simulink model "Pulsar_KTR_UBR"  (R2023b)
settings: Solver=VariableStepAuto  StartTime=0.0  StopTime=10  RelTol=1e-3
values from neighbouring files (symbols this model uses):
  itkip = [2411 2135 2015 2000 2055 2098 1860 1788 1659 1468 1423 1334 ... (23 elements, 23x1)]    [matlabubr.mat]
  zamanp = [0.1 0.2 0.3 0.4 0.5 1 1.5 2 2.5 3 3.25 3.35 ... (23 elements, 23x1)]    [matlabubr.mat]
undefined symbols (not defined in the file or in its folder): magnitude
libraries: simulink x1
settings Model: Creator=atzml  LastModifiedBy=atzml
settings OptimizationCC: BlockReduction=off  DefaultParameterBehavior=Inlined  BufferReuse=off

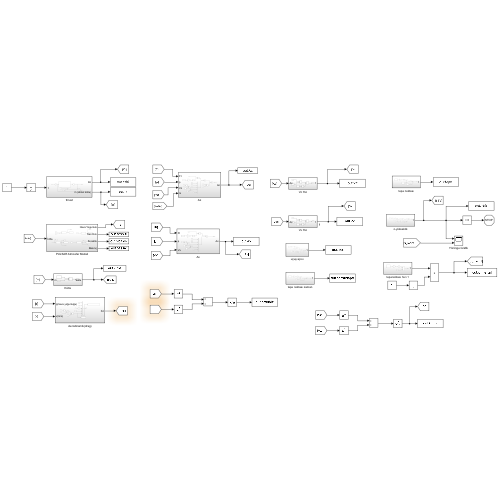
[thumbnail: Simulink's stored preview of the top-level diagram]
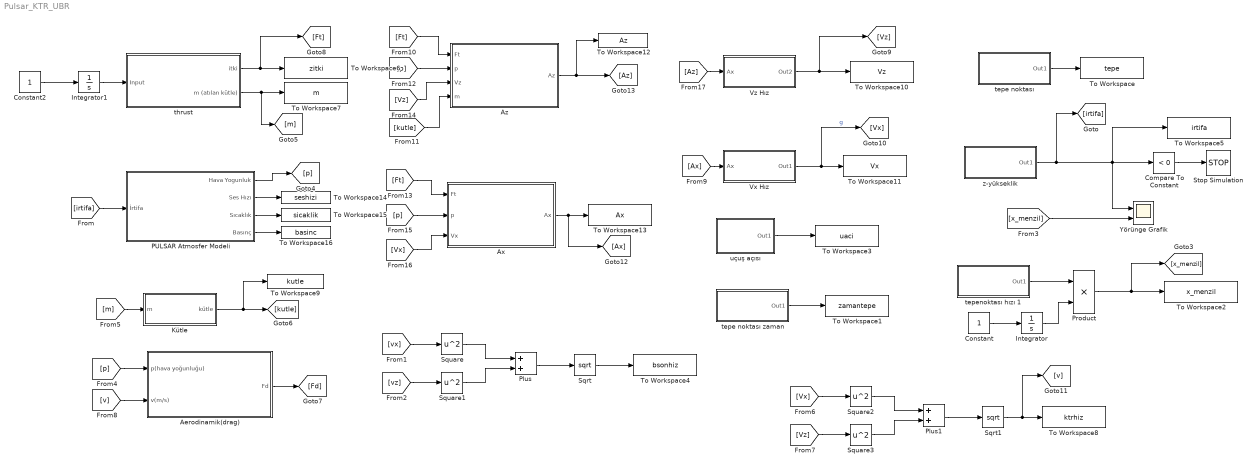
== system Pulsar_KTR_UBR ==
  Aerodinamik(drag) : Subsystem
  Ax : Subsystem
  Az : Subsystem
  Compare To Constant : simulink/Logic and Bit Operations/Compare To Constant  relop=<  const=0  OutDataTypeStr=boolean
  Constant : Constant
  Constant2 : Constant
  Integrator : Integrator
  Integrator1 : Integrator
  Kütle : Subsystem
  PULSAR Atmosfer Modeli : Subsystem
  Plus : Sum
  Plus1 : Sum
  Product : Product
  Sqrt : Sqrt
  Sqrt1 : Sqrt
  Square{,1..3} (4 alike) : Math  Operator=square
  Stop Simulation : Stop
  To Workspace : ToWorkspace  VariableName=tepe  SaveFormat=Timeseries  SampleTime=-1
  To Workspace1 : ToWorkspace  VariableName=zamantepe  SaveFormat=Timeseries  SampleTime=-1
  To Workspace10 : ToWorkspace  VariableName=Vz  SaveFormat=Timeseries  SampleTime=-1
  To Workspace11 : ToWorkspace  VariableName=Vx  SaveFormat=Timeseries  SampleTime=-1
  To Workspace12 : ToWorkspace  VariableName=Az  SaveFormat=Timeseries  SampleTime=-1
  To Workspace13 : ToWorkspace  VariableName=Ax  SaveFormat=Timeseries  SampleTime=-1
  To Workspace14 : ToWorkspace  VariableName=seshizi  SaveFormat=Timeseries  SampleTime=-1
  To Workspace15 : ToWorkspace  VariableName=sicaklik  SaveFormat=Timeseries  SampleTime=-1
  To Workspace16 : ToWorkspace  VariableName=basinc  SaveFormat=Timeseries  SampleTime=-1
  To Workspace2 : ToWorkspace  VariableName=x_menzil  SaveFormat=Timeseries  SampleTime=-1
  To Workspace3 : ToWorkspace  VariableName=uaci  SaveFormat=Timeseries  SampleTime=-1
  To Workspace4 : ToWorkspace  VariableName=bsonhiz  SaveFormat=Timeseries  SampleTime=-1
  To Workspace5 : ToWorkspace  VariableName=irtifa  SaveFormat=Timeseries  SampleTime=-1
  To Workspace6 : ToWorkspace  VariableName=zitki  SampleTime=-1
  To Workspace7 : ToWorkspace  VariableName=m  SaveFormat=Timeseries  SampleTime=-1
  To Workspace8 : ToWorkspace  VariableName=ktrhiz  SaveFormat=Timeseries  SampleTime=-1
  To Workspace9 : ToWorkspace  VariableName=kutle  SaveFormat=Timeseries  SampleTime=-1
  Vx Hız : Subsystem
  Vz Hız : Subsystem
  Yörünge Grafik : Scope  NumInputPorts=2
  tepe noktası : Subsystem
  tepe noktası zaman : Subsystem
  tepenoktası hızı 1 : Subsystem
  thrust : Subsystem
  uçuş açısı : Subsystem
  z-yükseklik : Subsystem
  wires:
  Compare To Constant/1 -> Stop Simulation/1
  Plus/1 -> Sqrt/1
  Constant/1 -> Integrator/1
  Square/1 -> Plus/1
  tepe noktası/1(Out1) -> To Workspace/1
  [x_menzil] -> Yörünge Grafik/2
  z-yükseklik/1(Out1) -> [irtifa], Yörünge Grafik/1, Compare To Constant/1, To Workspace5/1
  Integrator/1 -> Product/2
  Sqrt/1 -> To Workspace4/1
  Product/1 -> [x_menzil], To Workspace2/1
  tepenoktası hızı 1/1(Out1) -> Product/1
  [vz] -> Square1/1
  [vx] -> Square/1
  Square1/1 -> Plus/2
  tepe noktası zaman/1(Out1) -> To Workspace1/1
  uçuş açısı/1(Out1) -> To Workspace3/1
  [irtifa] -> PULSAR Atmosfer Modeli/1(İrtifa)
  PULSAR Atmosfer Modeli/1(Hava Yogunluk) -> [p]
  [p] -> Aerodinamik(drag)/1(p(hava yoğunluğu))
  [v] -> Aerodinamik(drag)/2(v(m/s))
  Aerodinamik(drag)/1(Fd) -> [Fd]
  thrust/2(m (atılan kütle)) -> [m], To Workspace7/1
  thrust/1(itki) -> [Ft], To Workspace6/1
  Constant2/1 -> Integrator1/1
  [m] -> Kütle/1(m)
  Kütle/1(kütle) -> To Workspace9/1, [kutle]
  Integrator1/1 -> thrust/1(Input)
  Vx Hız/1(Out1) -> To Workspace11/1, [Vx]  "g"
  Vz Hız/1(Out2) -> To Workspace10/1, [Vz]
  [Ft] -> Az/1(Ft)
  [kutle] -> Az/4(m)
  [p] -> Az/2(p)
  [p] -> Ax/2(p)
  [Ft] -> Ax/1(Ft)
  [Vz] -> Az/3(Vz)
  [Vx] -> Ax/3(Vx)
  Plus1/1 -> Sqrt1/1
  Sqrt1/1 -> [v], To Workspace8/1
  [Vx] -> Square2/1
  [Vz] -> Square3/1
  Square3/1 -> Plus1/2
  Square2/1 -> Plus1/1
  Ax/1(Ax) -> To Workspace13/1, [Ax]
  [Ax] -> Vx Hız/1(Ax)
  Az/1(Az) -> To Workspace12/1, [Az]
  [Az] -> Vz Hız/1(Ax)
  PULSAR Atmosfer Modeli/2(Ses Hızı) -> To Workspace14/1
  PULSAR Atmosfer Modeli/3(Sıcaklık) -> To Workspace15/1
  PULSAR Atmosfer Modeli/4(Basınç) -> To Workspace16/1

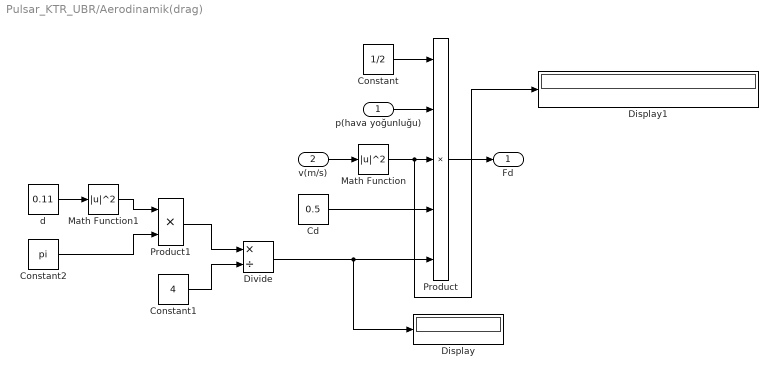
== system Pulsar_KTR_UBR/Aerodinamik(drag) ==
  p(hava yoğunluğu) : Inport
  v(m/s) : Inport  Port=2
  Cd : Constant  Value=0.5
  Constant : Constant  Value=1/2
  Constant1 : Constant  Value=4
  Constant2 : Constant  Value=pi
  Display : Display
  Display1 : Display
  Divide : Product  Inputs=*/
  Math Function : Math  Operator=magnitude^2
  Math Function1 : Math  Operator=magnitude^2
  Product : Product  Inputs=5
  Product1 : Product
  d : Constant  Value=0.11
  Fd : Outport
  wires:
  v(m/s)/1 -> Math Function/1
  Constant/1 -> Product/1
  p(hava yoğunluğu)/1 -> Product/2
  Math Function/1 -> Display1/1, Product/3
  Product/1 -> Fd/1
  Cd/1 -> Product/4
  Divide/1 -> Display/1, Product/5
  d/1 -> Math Function1/1
  Constant2/1 -> Product1/2
  Math Function1/1 -> Product1/1
  Product1/1 -> Divide/1
  Constant1/1 -> Divide/2

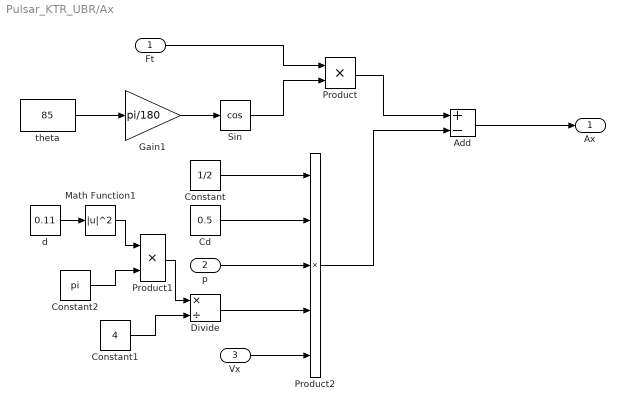
== system Pulsar_KTR_UBR/Ax ==
  Ft : Inport
  p : Inport  Port=2
  Vx : Inport  Port=3
  Add : Sum  Inputs=+-
  Cd : Constant  Value=0.5
  Constant : Constant  Value=1/2
  Constant1 : Constant  Value=4
  Constant2 : Constant  Value=pi
  Divide : Product  Inputs=*/
  Gain1 : Gain  Gain=pi/180
  Math Function1 : Math  Operator=magnitude^2
  Product : Product
  Product1 : Product
  Product2 : Product  Inputs=5
  Sin : Trigonometry  Operator=cos
  d : Constant  Value=0.11
  theta : Constant  Value=85
  Ax : Outport
  wires:
  Gain1/1 -> Sin/1
  theta/1 -> Gain1/1
  Ft/1 -> Product/1
  Sin/1 -> Product/2
  d/1 -> Math Function1/1
  Product1/1 -> Divide/1
  Constant1/1 -> Divide/2
  Constant2/1 -> Product1/2
  Math Function1/1 -> Product1/1
  Product/1 -> Add/1
  Constant/1 -> Product2/1
  Cd/1 -> Product2/2
  p/1 -> Product2/3
  Divide/1 -> Product2/4
  Product2/1 -> Add/2
  Vx/1 -> Product2/5
  Add/1 -> Ax/1

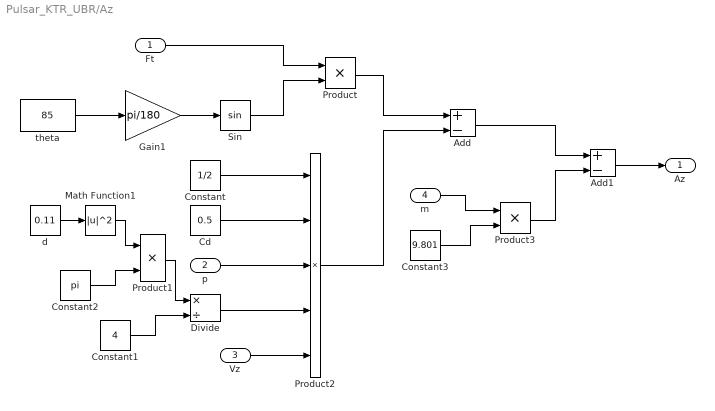
== system Pulsar_KTR_UBR/Az ==
  Ft : Inport
  p : Inport  Port=2
  Vz : Inport  Port=3
  m : Inport  Port=4
  Add : Sum  Inputs=+-
  Add1 : Sum  Inputs=+-
  Cd : Constant  Value=0.5
  Constant : Constant  Value=1/2
  Constant1 : Constant  Value=4
  Constant2 : Constant  Value=pi
  Constant3 : Constant  Value=9.801
  Divide : Product  Inputs=*/
  Gain1 : Gain  Gain=pi/180
  Math Function1 : Math  Operator=magnitude^2
  Product : Product
  Product1 : Product
  Product2 : Product  Inputs=5
  Product3 : Product
  Sin : Trigonometry
  d : Constant  Value=0.11
  theta : Constant  Value=85
  Az : Outport
  wires:
  Gain1/1 -> Sin/1
  theta/1 -> Gain1/1
  Ft/1 -> Product/1
  Sin/1 -> Product/2
  d/1 -> Math Function1/1
  Product1/1 -> Divide/1
  Constant1/1 -> Divide/2
  Constant2/1 -> Product1/2
  Math Function1/1 -> Product1/1
  Product/1 -> Add/1
  Constant/1 -> Product2/1
  Cd/1 -> Product2/2
  p/1 -> Product2/3
  Divide/1 -> Product2/4
  Product2/1 -> Add/2
  Vz/1 -> Product2/5
  m/1 -> Product3/1
  Constant3/1 -> Product3/2
  Add/1 -> Add1/1
  Product3/1 -> Add1/2
  Add1/1 -> Az/1

== system Pulsar_KTR_UBR/Kütle ==
  m : Inport
  Add : Sum
  Constant : Constant  Value=21.649
  kütle : Outport
  wires:
  m/1 -> Add/2
  Constant/1 -> Add/1
  Add/1 -> kütle/1

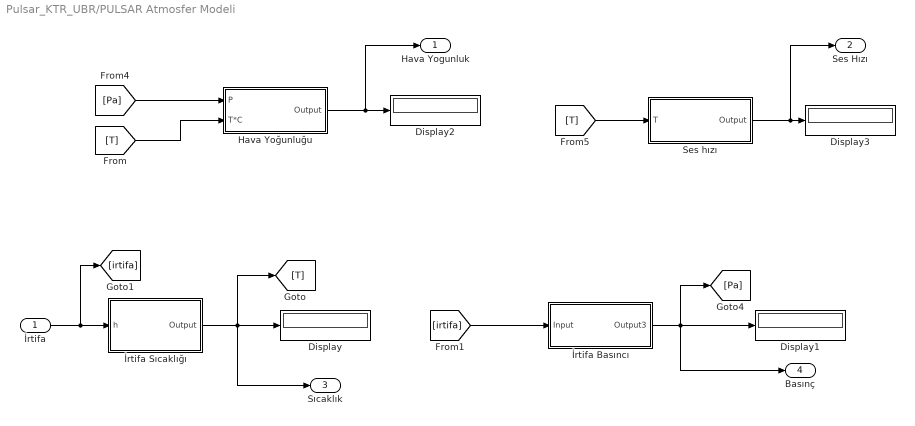
== system Pulsar_KTR_UBR/PULSAR Atmosfer Modeli ==
  İrtifa : Inport
  Display{,1..3} (4 alike) : Display
  Hava Yoğunluğu : Subsystem
  Ses hızı : Subsystem
  İrtifa Basıncı : Subsystem
  İrtifa Sıcaklığı : Subsystem
  Hava Yogunluk : Outport
  Ses Hızı : Outport  Port=2
  Sıcaklık : Outport  Port=3
  Basınç : Outport  Port=4
  wires:
  [irtifa] -> İrtifa Basıncı/1(Input)
  Hava Yoğunluğu/1(Output) -> Hava Yogunluk/1, Display2/1
  İrtifa/1 -> [irtifa], İrtifa Sıcaklığı/1(h)
  Ses hızı/1(Output) -> Ses Hızı/1, Display3/1
  İrtifa Sıcaklığı/1(Output) -> Sıcaklık/1, Display/1, [T]
  [Pa] -> Hava Yoğunluğu/1(P)
  İrtifa Basıncı/1(Output3) -> Basınç/1, Display1/1, [Pa]
  [T] -> Ses hızı/1(T)
  [T] -> Hava Yoğunluğu/2(T*C)

== system Pulsar_KTR_UBR/Vx Hız ==
  Ax : Inport
  Add : Sum
  Constant : Constant
  Integrator : Integrator
  Product : Product
  V0 : Constant  Value=2
  Out1 : Outport
  wires:
  V0/1 -> Add/2
  Ax/1 -> Add/1
  Add/1 -> Product/1
  Constant/1 -> Integrator/1
  Integrator/1 -> Product/2
  Product/1 -> Out1/1

== system Pulsar_KTR_UBR/Vz Hız ==
  Ax : Inport
  Add : Sum
  Constant : Constant
  Integrator : Integrator
  Product : Product
  V0 : Constant  Value=2
  Out2 : Outport
  wires:
  Constant/1 -> Integrator/1
  Product/1 -> Out2/1
  V0/1 -> Add/2
  Ax/1 -> Add/1
  Add/1 -> Product/1
  Integrator/1 -> Product/2

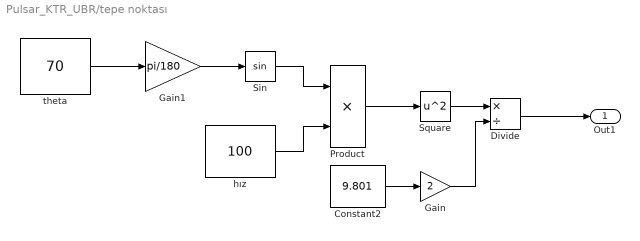
== system Pulsar_KTR_UBR/tepe noktası ==
  Constant2 : Constant  Value=9.801
  Divide : Product  Inputs=*/
  Gain : Gain  Gain=2
  Gain1 : Gain  Gain=pi/180
  Product : Product
  Sin : Trigonometry
  Square : Math  Operator=square
  hız : Constant  Value=100
  theta : Constant  Value=70
  Out1 : Outport
  wires:
  Sin/1 -> Product/1
  hız/1 -> Product/2
  Product/1 -> Square/1
  Square/1 -> Divide/1
  Constant2/1 -> Gain/1
  Gain/1 -> Divide/2
  Divide/1 -> Out1/1
  theta/1 -> Gain1/1
  Gain1/1 -> Sin/1

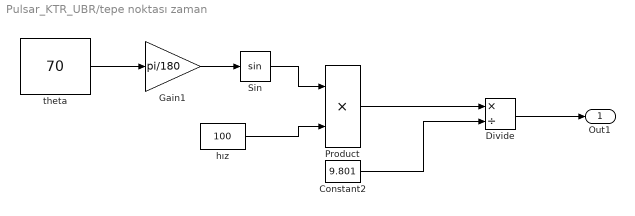
== system Pulsar_KTR_UBR/tepe noktası zaman ==
  Constant2 : Constant  Value=9.801
  Divide : Product  Inputs=*/
  Gain1 : Gain  Gain=pi/180
  Product : Product
  Sin : Trigonometry
  hız : Constant  Value=100
  theta : Constant  Value=70
  Out1 : Outport
  wires:
  Divide/1 -> Out1/1
  hız/1 -> Product/2
  Product/1 -> Divide/1
  Constant2/1 -> Divide/2
  Sin/1 -> Product/1
  Gain1/1 -> Sin/1
  theta/1 -> Gain1/1

== system Pulsar_KTR_UBR/tepenoktası hızı 1 ==
  Gain1 : Gain  Gain=pi/180
  Product : Product
  Sin : Trigonometry  Operator=cos
  hız : Constant  Value=100
  theta : Constant  Value=70
  Out1 : Outport
  wires:
  theta/1 -> Gain1/1
  Gain1/1 -> Sin/1
  hız/1 -> Product/2
  Sin/1 -> Product/1
  Product/1 -> Out1/1  "yatay hız"

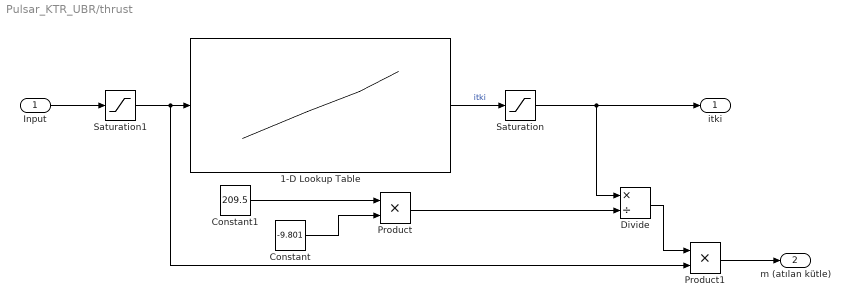
== system Pulsar_KTR_UBR/thrust ==
  Input : Inport
  1-D Lookup Table : Lookup_n-D  NumberOfTableDimensions=1  BreakpointsForDimension1=zamanp  Table=itkip  InternalRulePriority=Speed  RndMeth=Simplest
  Constant : Constant  Value=-9.801
  Constant1 : Constant  Value=209.5
  Divide : Product  Inputs=*/
  Product : Product
  Product1 : Product
  Saturation : Saturate  UpperLimit=3700  LowerLimit=0
  Saturation1 : Saturate  UpperLimit=6.5  LowerLimit=0
  itki : Outport
  m (atılan kütle) : Outport  Port=2
  wires:
  Constant/1 -> Product/2
  Constant1/1 -> Product/1
  Product/1 -> Divide/2
  Divide/1 -> Product1/1
  Product1/1 -> m (atılan kütle)/1
  Saturation/1 -> Divide/1, itki/1
  1-D Lookup Table/1 -> Saturation/1  "itki"
  Saturation1/1 -> Product1/2, 1-D Lookup Table/1
  Input/1 -> Saturation1/1

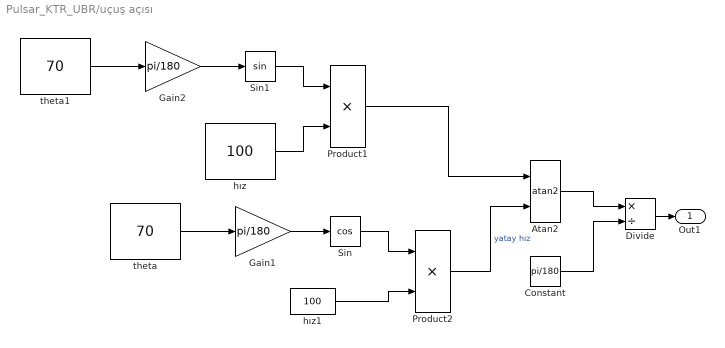
== system Pulsar_KTR_UBR/uçuş açısı ==
  Atan2 : Trigonometry  Operator=atan2
  Constant : Constant  Value=pi/180
  Divide : Product  Inputs=*/
  Gain1 : Gain  Gain=pi/180
  Gain2 : Gain  Gain=pi/180
  Product1 : Product
  Product2 : Product
  Sin : Trigonometry  Operator=cos
  Sin1 : Trigonometry
  hız : Constant  Value=100
  hız1 : Constant  Value=100
  theta : Constant  Value=70
  theta1 : Constant  Value=70
  Out1 : Outport
  wires:
  Atan2/1 -> Divide/1
  theta/1 -> Gain1/1
  Sin1/1 -> Product1/1
  hız1/1 -> Product2/2
  Gain2/1 -> Sin1/1
  theta1/1 -> Gain2/1
  Gain1/1 -> Sin/1
  Sin/1 -> Product2/1
  hız/1 -> Product1/2
  Product1/1 -> Atan2/1
  Constant/1 -> Divide/2
  Product2/1 -> Atan2/2  "yatay hız"
  Divide/1 -> Out1/1

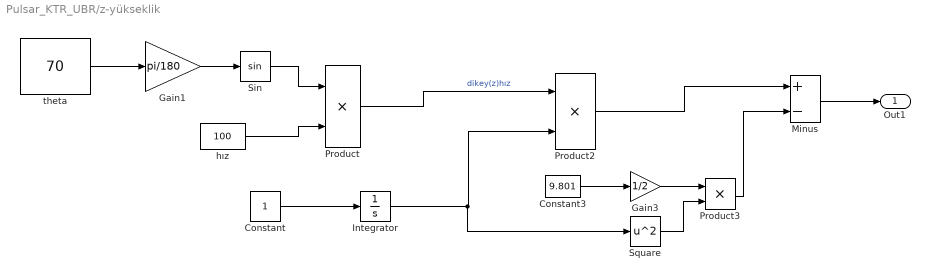
== system Pulsar_KTR_UBR/z-yükseklik ==
  Constant : Constant
  Constant3 : Constant  Value=9.801
  Gain1 : Gain  Gain=pi/180
  Gain3 : Gain  Gain=1/2
  Integrator : Integrator
  Minus : Sum  Inputs=+-
  Product : Product
  Product2 : Product
  Product3 : Product
  Sin : Trigonometry
  Square : Math  Operator=square
  hız : Constant  Value=100
  theta : Constant  Value=70
  Out1 : Outport
  wires:
  Product/1 -> Product2/1  "dikey(z)hız"
  Sin/1 -> Product/1
  hız/1 -> Product/2
  Gain1/1 -> Sin/1
  theta/1 -> Gain1/1
  Constant3/1 -> Gain3/1
  Integrator/1 -> Square/1, Product2/2
  Square/1 -> Product3/2
  Gain3/1 -> Product3/1
  Product3/1 -> Minus/2
  Product2/1 -> Minus/1
  Constant/1 -> Integrator/1
  Minus/1 -> Out1/1

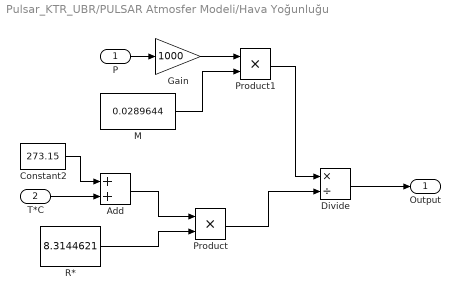
== system Pulsar_KTR_UBR/PULSAR Atmosfer Modeli/Hava Yoğunluğu ==
  P : Inport
  T*C : Inport  Port=2
  Add : Sum
  Constant2 : Constant  Value=273.15
  Divide : Product  Inputs=*/
  Gain : Gain  Gain=1000
  M : Constant  Value=0.0289644
  Product : Product
  Product1 : Product
  R* : Constant  Value=8.3144621
  Output : Outport
  wires:
  M/1 -> Product1/2
  R*/1 -> Product/2
  Divide/1 -> Output/1
  P/1 -> Gain/1
  Constant2/1 -> Add/1
  Product/1 -> Divide/2
  Product1/1 -> Divide/1
  Gain/1 -> Product1/1
  T*C/1 -> Add/2
  Add/1 -> Product/1

== system Pulsar_KTR_UBR/PULSAR Atmosfer Modeli/Ses hızı ==
  T : Inport
  Add : Sum
  Constant : Constant  Value=1.40
  Constant2 : Constant  Value=273.15
  Product : Product  Inputs=3
  R_sp : Constant  Value=287.052
  Sqrt : Sqrt
  Output : Outport
  wires:
  Constant2/1 -> Add/1
  T/1 -> Add/2
  Constant/1 -> Product/1
  R_sp/1 -> Product/2
  Add/1 -> Product/3
  Product/1 -> Sqrt/1
  Sqrt/1 -> Output/1

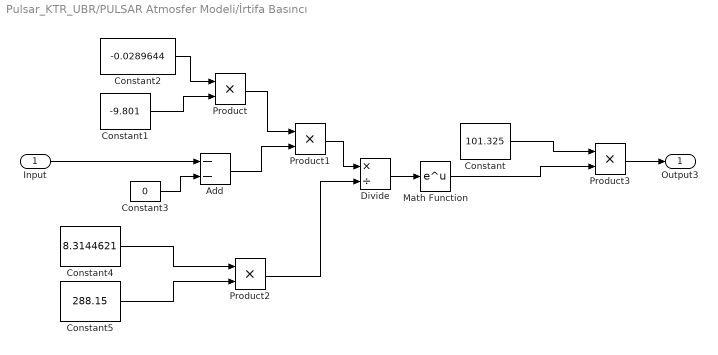
== system Pulsar_KTR_UBR/PULSAR Atmosfer Modeli/İrtifa Basıncı ==
  Input : Inport
  Add : Sum  Inputs=--
  Constant : Constant  Value=101.325
  Constant1 : Constant  Value=-9.801
  Constant2 : Constant  Value=-0.0289644
  Constant3 : Constant  Value=0
  Constant4 : Constant  Value=8.3144621
  Constant5 : Constant  Value=288.15
  Divide : Product  Inputs=*/
  Math Function : Math
  Product{,1..3} (4 alike) : Product
  Output3 : Outport
  wires:
  Constant2/1 -> Product/1
  Constant1/1 -> Product/2
  Input/1 -> Add/1
  Constant3/1 -> Add/2
  Add/1 -> Product1/2
  Product/1 -> Product1/1
  Constant4/1 -> Product2/1
  Constant5/1 -> Product2/2
  Product1/1 -> Divide/1
  Product2/1 -> Divide/2
  Divide/1 -> Math Function/1
  Constant/1 -> Product3/1
  Math Function/1 -> Product3/2
  Product3/1 -> Output3/1

== system Pulsar_KTR_UBR/PULSAR Atmosfer Modeli/İrtifa Sıcaklığı ==
  h : Inport
  Add : Sum  Inputs=--
  Add1 : Sum
  Product1 : Product
  atlama : Constant  Value=0.0065
  galtitude : Constant  Value=0
  tsıcaklık : Constant  Value=15
  Output : Outport
  wires:
  Product1/1 -> Add1/1
  galtitude/1 -> Add/2
  Add1/1 -> Output/1
  Add/1 -> Product1/2
  tsıcaklık/1 -> Add1/2
  h/1 -> Add/1
  atlama/1 -> Product1/1
